simulink library "MotionSimPlanarLibrary"  (Simulink 7.8)
settings: Solver=ode45  StartTime=0.0  StopTime=10.0  RelTol=1e-3
values from neighbouring files (symbols this model uses):
  sysmodel = CalcDof( sysmodel)    [conv2simulink.m]
undefined symbols (not defined in the file or in its folder): selectnum
settings Model: Creator=john  LastModifiedBy=john

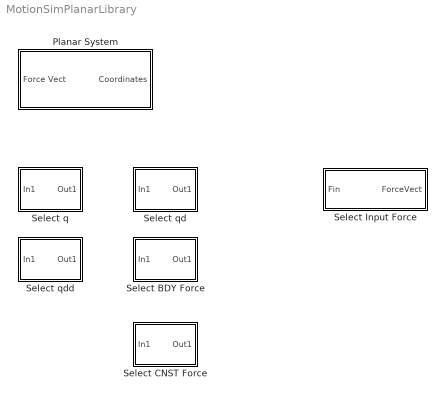
== system MotionSimPlanarLibrary ==
  Planar System : Subsystem
  Select BDY Force : Subsystem  AncestorBlock=MotionSimPlanarLibrary/Select BDY Force  mask{Bodynum=3, Selectnum=Fx}
      mask prompts: Bodynum "Body Number"; Selectnum "Select Coordinate"
      mask StyleString: edit,popup(Fx|Fy|Tz)
      mask Display:
      | port_label('input',1,'coord');
      | port_label('output',1,'Fn');
  Select CNST Force : Subsystem  AncestorBlock=MotionSimPlanarLibrary/Select CNST Force  mask{Bodynum=2, Selectnum=Fx}
      mask prompts: Bodynum "Body Number"; Selectnum "Select Coordinate"
      mask StyleString: edit,popup(Fx|Fy|Tz)
      mask Display:
      | port_label('input',1,'coord');
      | port_label('output',1,'Fn');
  Select Input Force : Subsystem  mask{BodyNum=1, ForceNum=Tx}
      mask prompts: BodyNum "Body Number"; ForceNum "Force"
      mask StyleString: edit,popup(Fx|Fy|Fz|Tx|Ty|Tz)
  Select q : Subsystem  AncestorBlock=MotionSimPlanarLibrary/Select q  mask{Bodynum=2, Selectnum=X}
      mask prompts: Bodynum "Body Number"; Selectnum "Select Coordinate"
      mask StyleString: edit,popup(X|Y|PHI)
      mask Display:
      | port_label('input',1,'coord');
      | port_label('output',1,'q');
  Select qd : Subsystem  AncestorBlock=MotionSimPlanarLibrary/Select qd  mask{Bodynum=2, Selectnum=Xd}
      mask prompts: Bodynum "Body Number"; Selectnum "Select Coordinate"
      mask StyleString: edit,popup(Xd|Yd|PHId)
      mask Display:
      | port_label('input',1,'coord');
      | port_label('output',1,'qd');
  Select qdd : Subsystem  AncestorBlock=MotionSimPlanarLibrary/Select qdd  mask{Bodynum=2, Selectnum=Xdd}
      mask prompts: Bodynum "Body Number"; Selectnum "Select Coordinate"
      mask StyleString: edit,popup(Xdd|Ydd|PHIdd)
      mask Display:
      | port_label('input',1,'coord');
      | port_label('output',1,'qdd');

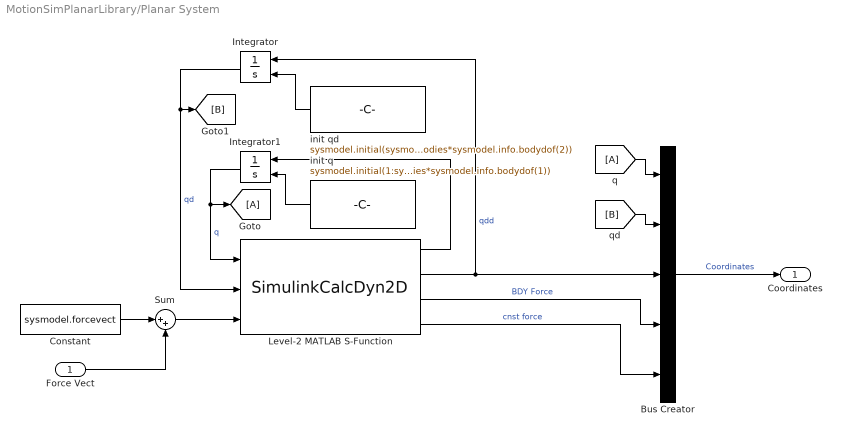
== system MotionSimPlanarLibrary/Planar System ==
  Force Vect : Inport
  Bus Creator : BusCreator  Inputs=5
  Constant : Constant  Value=sysmodel.forcevect
  Integrator : Integrator  InitialConditionSource=external
  Integrator1 : Integrator  InitialConditionSource=external
  Level-2 MATLAB S-Function : M-S-Function  FunctionName=SimulinkCalcDyn2D  Parameters=sysmodel
      mask Display:
      | port_label('output',1,'qd');
      | port_label('output',2,'qdd');
      | port_label('output',3,'Body Forces');
      | port_label('output',4,'Constraint Forces');
      | 
      | port_label('input',1,'q');
      | port_label('input',2,'qd');
  Sum : Sum  Inputs=|++
  init q : Constant  Value=sysmodel.initial(1:sysmodel.info.bodies*sysmodel.info.bodydof(1))
  init qd : Constant  Value=sysmodel.initial(sysmodel.info.bodies*sysmodel.info.bodydof(1)+1:sysmodel.info.bodies*sysmodel.info.bodydof(1)+sysmodel.info.bodies*sysmodel.info.bodydof(2))
  Coordinates : Outport
  wires:
  Bus Creator/1 -> Coordinates/1  "Coordinates"
  [B] -> Bus Creator/2
  [A] -> Bus Creator/1
  Constant/1 -> Sum/1
  Force Vect/1 -> Sum/2
  Sum/1 -> Level-2 MATLAB S-Function/3
  Level-2 MATLAB S-Function/4 -> Bus Creator/5  "cnst force"
  Level-2 MATLAB S-Function/3 -> Bus Creator/4  "BDY Force"
  init qd/1 -> Integrator/2
  init q/1 -> Integrator1/2
  Level-2 MATLAB S-Function/2 -> Bus Creator/3, Integrator/1  "qdd"
  Level-2 MATLAB S-Function/1 -> Integrator1/1
  Integrator/1 -> [B], Level-2 MATLAB S-Function/2  "qd"
  Integrator1/1 -> [A], Level-2 MATLAB S-Function/1  "q"

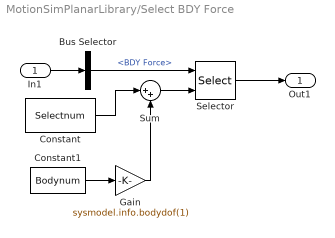
== system MotionSimPlanarLibrary/Select BDY Force ==
  In1 : Inport
  Bus Selector : BusSelector  OutputSignals=BDY Force
  Constant : Constant  Value=Selectnum
  Constant1 : Constant  Value=Bodynum
  Gain : Gain  Gain=sysmodel.info.bodydof(1)
  Selector : Selector  InputPortWidth=sysmodel.info.bodies*sysmodel.info.bodydof(1)  IndexOptions=Index vector (port)  Indices=[Bodynum+selectnum]  OutputSizes=1
  Sum : Sum  Inputs=|++
  Out1 : Outport
  wires:
  Bus Selector/1 -> Selector/1  "<BDY Force>"
  In1/1 -> Bus Selector/1
  Gain/1 -> Sum/2
  Constant/1 -> Sum/1
  Sum/1 -> Selector/2
  Constant1/1 -> Gain/1
  Selector/1 -> Out1/1

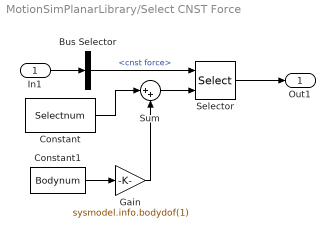
== system MotionSimPlanarLibrary/Select CNST Force ==
  In1 : Inport
  Bus Selector : BusSelector  OutputSignals=cnst force
  Constant : Constant  Value=Selectnum
  Constant1 : Constant  Value=Bodynum
  Gain : Gain  Gain=sysmodel.info.bodydof(1)
  Selector : Selector  InputPortWidth=sysmodel.info.bodies*sysmodel.info.bodydof(1)  IndexOptions=Index vector (port)  Indices=[Bodynum+selectnum]  OutputSizes=1
  Sum : Sum  Inputs=|++
  Out1 : Outport
  wires:
  Bus Selector/1 -> Selector/1  "<cnst force>"
  In1/1 -> Bus Selector/1
  Gain/1 -> Sum/2
  Constant/1 -> Sum/1
  Sum/1 -> Selector/2
  Constant1/1 -> Gain/1
  Selector/1 -> Out1/1

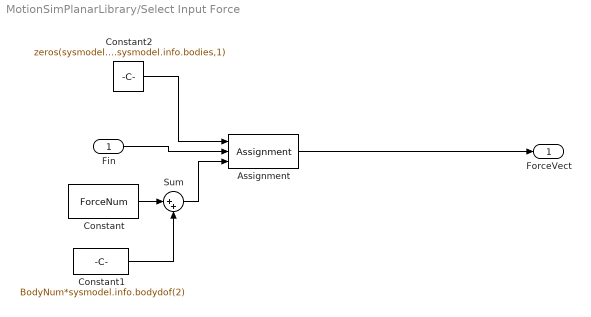
== system MotionSimPlanarLibrary/Select Input Force ==
  Fin : Inport
  Assignment : Assignment  IndexOptions=Index vector (port)  Indices=9  OutputSizes=1
  Constant : Constant  Value=ForceNum
  Constant1 : Constant  Value=BodyNum*sysmodel.info.bodydof(2)
  Constant2 : Constant  Value=zeros(sysmodel.info.bodydof(2)*sysmodel.info.bodies,1)
  Sum : Sum  Inputs=|++
  ForceVect : Outport
  wires:
  Sum/1 -> Assignment/3
  Constant/1 -> Sum/1
  Constant1/1 -> Sum/2
  Fin/1 -> Assignment/2
  Constant2/1 -> Assignment/1
  Assignment/1 -> ForceVect/1

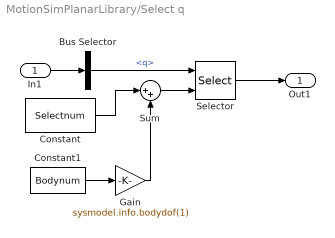
== system MotionSimPlanarLibrary/Select q ==
  In1 : Inport
  Bus Selector : BusSelector  OutputSignals=q
  Constant : Constant  Value=Selectnum
  Constant1 : Constant  Value=Bodynum
  Gain : Gain  Gain=sysmodel.info.bodydof(1)
  Selector : Selector  InputPortWidth=sysmodel.info.bodies*sysmodel.info.bodydof(1)  IndexOptions=Index vector (port)  Indices=[Bodynum+selectnum]  OutputSizes=1
  Sum : Sum  Inputs=|++
  Out1 : Outport
  wires:
  Bus Selector/1 -> Selector/1  "<q>"
  In1/1 -> Bus Selector/1
  Gain/1 -> Sum/2
  Constant/1 -> Sum/1
  Sum/1 -> Selector/2
  Constant1/1 -> Gain/1
  Selector/1 -> Out1/1

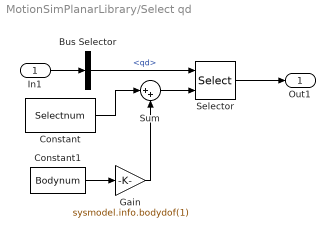
== system MotionSimPlanarLibrary/Select qd ==
  In1 : Inport
  Bus Selector : BusSelector  OutputSignals=qd
  Constant : Constant  Value=Selectnum
  Constant1 : Constant  Value=Bodynum
  Gain : Gain  Gain=sysmodel.info.bodydof(1)
  Selector : Selector  InputPortWidth=sysmodel.info.bodies*sysmodel.info.bodydof(1)  IndexOptions=Index vector (port)  Indices=[Bodynum+selectnum]  OutputSizes=1
  Sum : Sum  Inputs=|++
  Out1 : Outport
  wires:
  Bus Selector/1 -> Selector/1  "<qd>"
  In1/1 -> Bus Selector/1
  Gain/1 -> Sum/2
  Constant/1 -> Sum/1
  Sum/1 -> Selector/2
  Constant1/1 -> Gain/1
  Selector/1 -> Out1/1

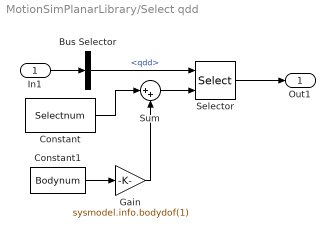
== system MotionSimPlanarLibrary/Select qdd ==
  In1 : Inport
  Bus Selector : BusSelector  OutputSignals=qdd
  Constant : Constant  Value=Selectnum
  Constant1 : Constant  Value=Bodynum
  Gain : Gain  Gain=sysmodel.info.bodydof(1)
  Selector : Selector  InputPortWidth=sysmodel.info.bodies*sysmodel.info.bodydof(1)  IndexOptions=Index vector (port)  Indices=[Bodynum+selectnum]  OutputSizes=1
  Sum : Sum  Inputs=|++
  Out1 : Outport
  wires:
  Bus Selector/1 -> Selector/1  "<qdd>"
  In1/1 -> Bus Selector/1
  Gain/1 -> Sum/2
  Constant/1 -> Sum/1
  Sum/1 -> Selector/2
  Constant1/1 -> Gain/1
  Selector/1 -> Out1/1
